simulink model "wind_turbine_control_improved_model"  (R2018a)
settings: Solver=ode4  StartTime=0.0  StopTime=15  FixedStep=10e-6  RelTol=1e-3
undefined symbols (not defined in the file): DiscIntNeverNeededParam
libraries: powerlib x7, powerlib_meascontrol x3, re_lib x1
settings Model: Creator=chaka  LastModifiedBy=chaka

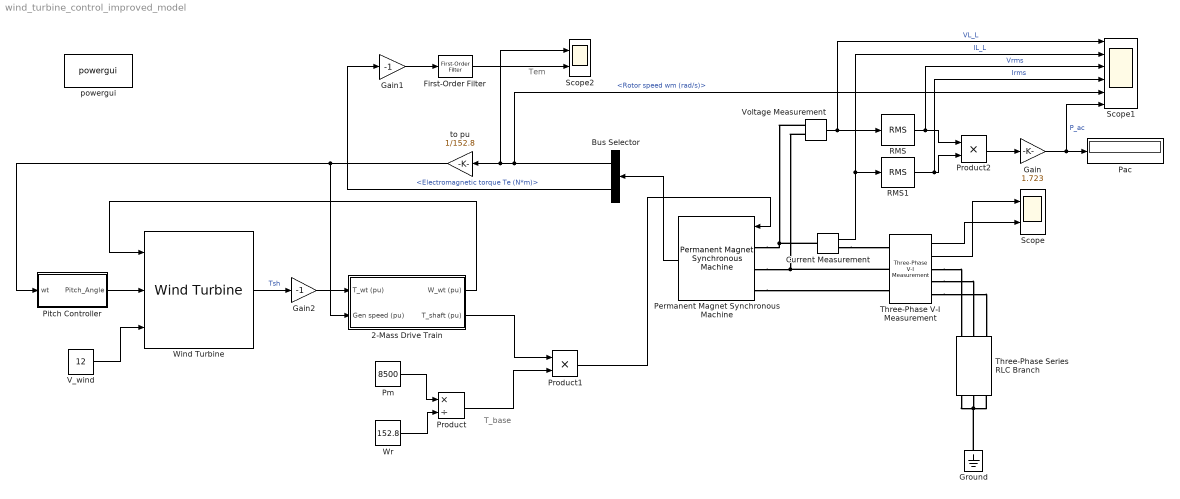
== system wind_turbine_control_improved_model ==
  note: Tem
  note: T_base
  2-Mass Drive Train : Subsystem
  Bus Selector : BusSelector  OutputSignals=Rotor speed wm (rad/s),Electromagnetic torque Te (N*m)
  Current Measurement : powerlib/Measurements/Current Measurement  PhasorSimulation=off  OutputType=Complex  PSBequivalent=0
  First-Order Filter : powerlib_meascontrol/Filters/First-Order Filter  FilterType=Lowpass  Tc=1e-3  Ts=50e-6  Initialize=on  Vac_Init=[0, 0, 50]  Vdc_Init=0  PlotResponse=off  FreqRange="[0,  200,  1]"
      settings: SourceProductName=Simscape Power Systems
  Gain : Gain  Gain=1.723
  Gain1 : Gain  Gain=-1
  Gain2 : Gain  Gain=-1
  Ground : powerlib/Elements/Ground  LConnTagsString=a
  Pac : Display
  Permanent Magnet Synchronous Machine : powerlib/Machines/Permanent Magnet Synchronous Machine  NbPhases=3  FluxDistribution=Sinusoidal  RotorType=Round  MechanicalLoad=Torque Tm  PresetModel=No  ShowDetailedParameters=on  MeasurementBus=off  Resistance=0.425  Inductance=8.5e-3  dqInductances=[8.5e-3,8.5e-3]  La=0.000395  MachineConstant=Flux linkage established by magnets (V.s)  Flux=0.433  VoltageCst=392.6876  TorqueCst=3.2475  Flat=120  Mechanical=[0.01197 0.001189 5 0]  PolePairs=4  InitialConditions=[0,0, 0,0]  InitialConditions5ph=[0 0 0 0 0 0]  TsPowergui=0  TsBlock=50e-6  RefAngle=90 degrees behind phase A axis (modified Park)
      settings: SourceProductName=Simscape Power Systems
  Pitch Controller : Subsystem
  Pm : Constant  Value=8500
  Product : Product  Inputs=*/
  Product1 : Product
  Product2 : Product
  RMS : powerlib_meascontrol/Measurements/RMS  TrueRMS=on  Freq=50  RMSInit=120  Ts=50e-6
  RMS1 : powerlib_meascontrol/Measurements/RMS  TrueRMS=on  Freq=50  RMSInit=120  Ts=50e-6
  Scope : Scope  NumInputPorts=2
  Scope1 : Scope  NumInputPorts=6
  Scope2 : Scope  NumInputPorts=2
  Three-Phase Series RLC Branch : powerlib/Elements/Three-Phase Series RLC Branch  LConnTagsString=A|B|C  RConnTagsString=A|B|C  BranchType=R  Resistance=1  Inductance=1e-3  Capacitance=1e-6  Measurements=None
  Three-Phase V-I Measurement : powerlib/Measurements/Three-Phase V-I Measurement  VoltageMeasurement=phase-to-phase  SetLabelV=off  LabelV=Vabc  Vpu=off  VpuLL=off  CurrentMeasurement=yes  SetLabelI=off  LabelI=Iabc  Ipu=off  Pbase=100e6  Vbase=500e3  OutputType=Complex  PhasorSimulation=off  PSBequivalent=0
  V_wind : Constant  Value=12
  Voltage Measurement : powerlib/Measurements/Voltage Measurement  PhasorSimulation=off  OutputType=Complex  PSBequivalent=0
  Wind Turbine : re_lib/Wind Generation/Wind Turbine  Pnom=8.5e3  Pelec_base=8.5e3/0.9  wind_base=12  P_wind_base=0.8  speed_nom=1  pitch_angle=0  c1_c6="[0.51763          116          0.4            5           21     0.006795]"  cp_nom=0.48  lambda_nom=8.1
      settings: SourceProductName=Simscape Power Systems  SourceProductBaseCode=PS
  Wr : Constant  Value=152.8
  powergui : powerlib/powergui  Priority=1  SimulationMode=Discrete  SampleTime=20e-6  frequency=60  Iterations=50  frequencyindice=0  Pbase=100e6  ErrMax=1e-4  UnitsV=kV  UnitsW=MW  buscounter=0  FunctionMessages=off  echomessages=off  EnableUseOfTLC=off  CurrentSourceSwitches=off  DisableSnubberDevices=off  DisableRonSwitches=off  DisableVfSwitches=off  DisplayEquations=off  SolverType=Tustin/Backward Euler (TBE)  Interpol=off  ExternalGateDelay=off  methode=off  Ts=100  x0status=blocks  SPID=on  SwTol=0  HookPort=off  RestoreLinks=warning  ResistiveCurrentMeasurement=off  Frange=[0:2:500]  Ylog=off  Xlog=on  ShowGrid=off  save=off  variable=ZData  structure=0  ZoomFFT=off  StartTime=0.0  cycles=1  DisplayStyle=1  fundamental=60  FreqAxis=off  MaxFrequency=1000  frequencyindicesteady=1  RmsSteady=1  display=off
  to pu : Gain  Gain=1/152.8
  wires:
  Pitch Controller/1(Pitch_Angle) -> Wind Turbine/2
  V_wind/1 -> Wind Turbine/3
  Wind Turbine/1 -> Gain2/1  "Tsh"
  Permanent Magnet Synchronous Machine/1 -> Bus Selector/1
  Bus Selector/1 -> Scope1/5, to pu/1, Scope2/1  "<Rotor speed wm (rad/s)>"
  to pu/1 -> Pitch Controller/1(wt), 2-Mass Drive Train/2(Gen speed (pu))
  2-Mass Drive Train/1(W_wt (pu)) -> Wind Turbine/1
  2-Mass Drive Train/2(T_shaft (pu)) -> Product1/1
  Product/1 -> Product1/2
  Pm/1 -> Product/1
  Wr/1 -> Product/2
  Product1/1 -> Permanent Magnet Synchronous Machine/1
  Three-Phase V-I Measurement/2 -> Scope/1
  Three-Phase V-I Measurement/1 -> Scope/2
  Voltage Measurement/1 -> RMS/1, Scope1/1  "VL_L"
  Current Measurement/1 -> RMS1/1, Scope1/2  "IL_L"
  RMS/1 -> Scope1/3, Product2/1  "Vrms"
  RMS1/1 -> Scope1/4, Product2/2  "Irms"
  Product2/1 -> Gain/1
  Gain/1 -> Scope1/6, Pac/1  "P_ac"
  Gain1/1 -> First-Order Filter/1
  Bus Selector/2 -> Gain1/1  "<Electromagnetic torque Te (N*m)>"
  First-Order Filter/1 -> Scope2/2
  Gain2/1 -> 2-Mass Drive Train/1(T_wt (pu))
  connections:
  Three-Phase Series RLC Branch/RConn1 -- Three-Phase Series RLC Branch/RConn2 -- Three-Phase Series RLC Branch/RConn3 -- Ground/LConn1
  Three-Phase V-I Measurement/RConn3 -- Three-Phase Series RLC Branch/LConn3
  Three-Phase V-I Measurement/RConn2 -- Three-Phase Series RLC Branch/LConn2
  Three-Phase V-I Measurement/RConn1 -- Three-Phase Series RLC Branch/LConn1
  Voltage Measurement/LConn1 -- Permanent Magnet Synchronous Machine/LConn1 -- Current Measurement/LConn1
  Three-Phase V-I Measurement/LConn2 -- Permanent Magnet Synchronous Machine/LConn2 -- Voltage Measurement/LConn2
  Permanent Magnet Synchronous Machine/LConn3 -- Three-Phase V-I Measurement/LConn3
  Current Measurement/RConn1 -- Three-Phase V-I Measurement/LConn1

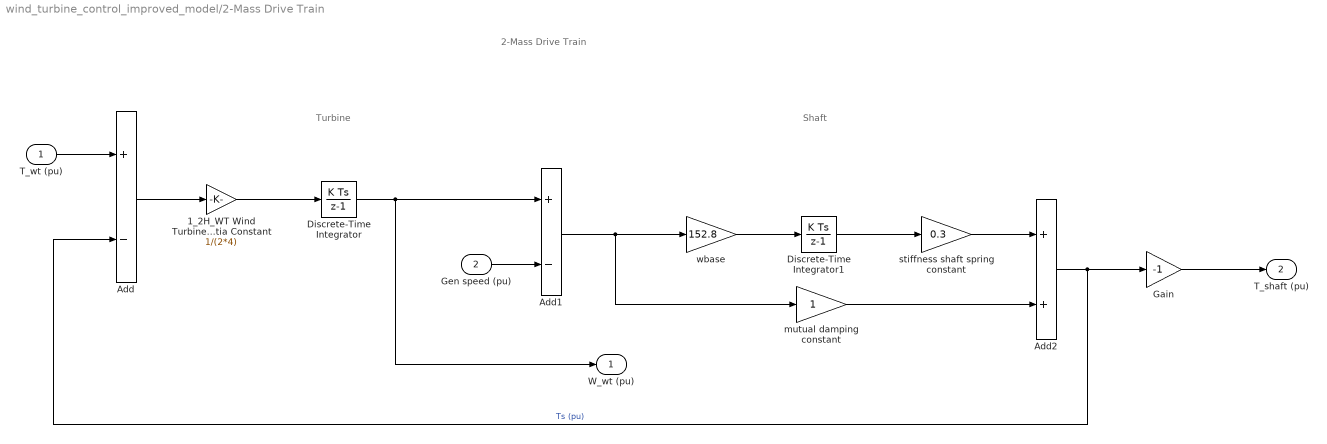
== system wind_turbine_control_improved_model/2-Mass Drive Train ==
  note: Turbine
  note: 2-Mass Drive Train
  note: Shaft
  T_wt (pu) : Inport
  Gen speed (pu) : Inport  Port=2
  1_2H_WT Wind Turbine Inertia Constant : Gain  Gain=1/(2*4)
  Add : Sum  Inputs=+-
  Add1 : Sum  Inputs=+-
  Add2 : Sum
  Discrete-Time Integrator : DiscreteIntegrator  SampleTime=-1  ICPrevOutput=DiscIntNeverNeededParam  ICPrevScaledInput=DiscIntNeverNeededParam
  Discrete-Time Integrator1 : DiscreteIntegrator  InitialCondition=1/0.3  SampleTime=50e-6  ICPrevOutput=DiscIntNeverNeededParam  ICPrevScaledInput=DiscIntNeverNeededParam
  Gain : Gain  Gain=-1
  mutual damping constant : Gain
  stiffness shaft spring constant : Gain  Gain=0.3
  wbase : Gain  Gain=152.8
  W_wt (pu) : Outport
  T_shaft (pu) : Outport  Port=2
  wires:
  T_wt (pu)/1 -> Add/1
  Add/1 -> 1_2H_WT Wind Turbine Inertia Constant/1
  1_2H_WT Wind Turbine Inertia Constant/1 -> Discrete-Time Integrator/1
  Discrete-Time Integrator/1 -> Add1/1, W_wt (pu)/1
  Gen speed (pu)/1 -> Add1/2
  Add1/1 -> mutual damping constant/1, wbase/1
  wbase/1 -> Discrete-Time Integrator1/1
  Discrete-Time Integrator1/1 -> stiffness shaft spring constant/1
  stiffness shaft spring constant/1 -> Add2/1
  mutual damping constant/1 -> Add2/2
  Add2/1 -> Gain/1, Add/2  "Ts (pu)"
  Gain/1 -> T_shaft (pu)/1

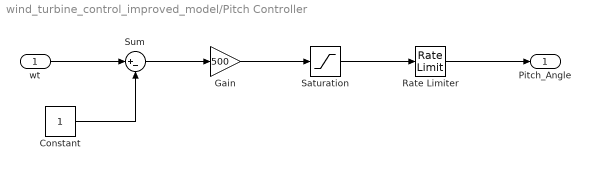
== system wind_turbine_control_improved_model/Pitch Controller ==
  wt : Inport
  Constant : Constant
  Gain : Gain  Gain=500
  Rate Limiter : RateLimiter  RisingSlewLimit=2  FallingSlewLimit=-2  SampleTimeMode=inherited
  Saturation : Saturate  UpperLimit=45  LowerLimit=0
  Sum : Sum  Inputs=|+-
  Pitch_Angle : Outport
  wires:
  wt/1 -> Sum/1
  Constant/1 -> Sum/2
  Sum/1 -> Gain/1
  Gain/1 -> Saturation/1
  Saturation/1 -> Rate Limiter/1
  Rate Limiter/1 -> Pitch_Angle/1
